simulink model "w3_p2"  (R2020b)
settings: Solver=FixedStepDiscrete  StartTime=0.0  StopTime=150  FixedStep=1  RelTol=1e-3
undefined symbols (not defined in the file): DiscIntNeverNeededParam
libraries: simulink x1
settings Model: Creator=mluser  LastModifiedBy=mluser

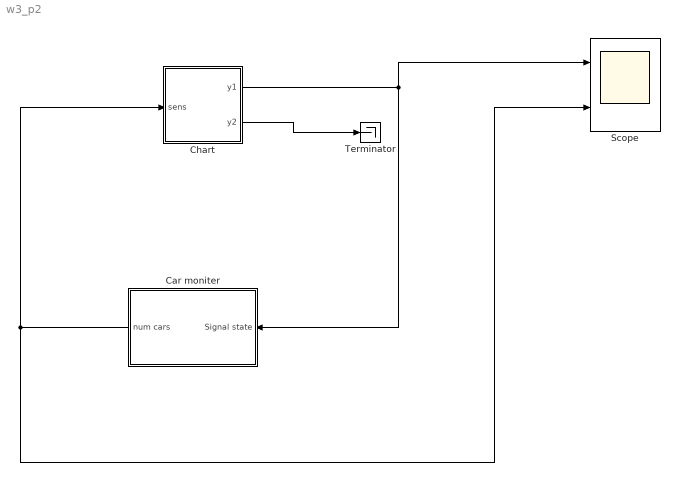
== system w3_p2 ==
  Car moniter : Subsystem
  Chart : Stateflow chart  TreatAsAtomicUnit=on
  Scope : Scope  NumInputPorts=2
  Terminator : Terminator
  wires:
  Chart/1(y1) -> Scope/1, Car moniter/1(Signal state)
  Car moniter/1(num cars) -> Chart/1(sens), Scope/2
  Chart/2(y2) -> Terminator/1

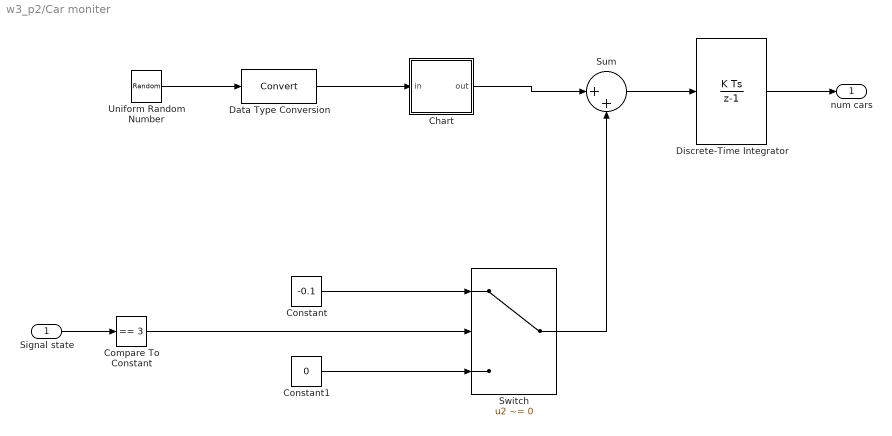
== system w3_p2/Car moniter ==
  Signal state : Inport
  Chart : Stateflow chart  TreatAsAtomicUnit=on
  Compare To Constant : simulink/Logic and Bit Operations/Compare To Constant  relop===  const=3  OutDataTypeStr=boolean
  Constant : Constant  Value=-0.1
  Constant1 : Constant  Value=0
  Data Type Conversion : DataTypeConversion
  Discrete-Time Integrator : DiscreteIntegrator  SampleTime=-1  LimitOutput=on  LowerSaturationLimit=0  ICPrevOutput=DiscIntNeverNeededParam  ICPrevScaledInput=DiscIntNeverNeededParam
  Sum : Sum  Inputs=|++
  Switch : Switch  Criteria=u2 ~= 0
  Uniform Random Number : UniformRandomNumber  Minimum=0  Maximum=100  Seed=177836  SampleTime=0
  num cars : Outport
  wires:
  Uniform Random Number/1 -> Data Type Conversion/1
  Switch/1 -> Sum/2
  Constant1/1 -> Switch/3
  Constant/1 -> Switch/1
  Compare To Constant/1 -> Switch/2
  Signal state/1 -> Compare To Constant/1
  Sum/1 -> Discrete-Time Integrator/1
  Discrete-Time Integrator/1 -> num cars/1
  Data Type Conversion/1 -> Chart/1(in)
  Chart/1(out) -> Sum/1

== stateflow chart w3_p2/Car moniter/Chart ==
  (default) -> (junction 1) : {out = in > 98;}
  data: in input; out output double

== stateflow chart w3_p2/Chart ==
  settings: stateMachineType=MOORE_MACHINE  initializeOutput=1
  state Stop
    y1 = RED;
    y2 = GREEN;
  state StopForTraffic
    y1 = RED;
    y2 = GREEN;
  state StopToGo
    y1 = RED;
    y2 = YELLOW;
  state GoToStop
    y1 = YELLOW;
    y2 = RED;
  state Go
    y1 = GREEN;
    y2 = RED;
  (default) -> Stop
  StopForTraffic -> StopToGo : [sens]
  Stop -> StopForTraffic : after(20,tick)
  GoToStop -> Stop : after (3,tick)
  StopToGo -> Go : after(3,tick)
  Go -> GoToStop : after(10,tick)
  data: sens input; y1 output double; y2 output double; GREEN constant double =3; RED constant double =1; YELLOW constant double =2
